simulink model "HINF4INDIFullLoop"  (R2021a)
settings: Solver=VariableStepAuto  StartTime=0.0  StopTime=50  RelTol=1e-3
values from neighbouring files (symbols this model uses):
  Ahg2 = blkdiag(Ahg2, Ahcg)    [HinFSynINDIFullLoop.m]
  Ahs3 = blkdiag(Ahs3, Ahcs)    [HinFSynINDIFullLoop.m]
  Ahs7 = blkdiag(Ahs7, Ahcs)    [HinFSynINDIFullLoop.m]
  Amc = d2c(Amd,'tustin')    [HinFSynINDIFullLoop.m]
  Asc = d2c(Asd,'tustin')    [HinFSynINDIFullLoop.m]
  Bhg2 = blkdiag(Bhg2, Bhcg)    [HinFSynINDIFullLoop.m]
  Bhs3 = blkdiag(Bhs3, Bhcs)    [HinFSynINDIFullLoop.m]
  Bhs7 = blkdiag(Bhs7, Bhcs)    [HinFSynINDIFullLoop.m]
  Chg2 = blkdiag(Chg2, Chcg)    [HinFSynINDIFullLoop.m]
  Chs3 = blkdiag(Chs3, Chcs)    [HinFSynINDIFullLoop.m]
  Chs7 = blkdiag(Chs7, Chcs)    [HinFSynINDIFullLoop.m]
  Dhg2 = blkdiag(Dhg2, Dhcg)    [HinFSynINDIFullLoop.m]
  Dhs3 = blkdiag(Dhs3, Dhcs)    [HinFSynINDIFullLoop.m]
  Dhs7 = blkdiag(Dhs7, Dhcs)    [HinFSynINDIFullLoop.m]
  Gs = [-10.67  10.67  0     0     0     0 0 ... (first row only)    [HinFSynINDIFullLoop.m]
  Gs_inv = pinv(Gs)    [HinFSynINDIFullLoop.m]
  Kdg = diag([2.0; 1.8])    [HinFSynINDIFullLoop.m]
  Kds = [10; 18; 18]    [HinFSynINDIFullLoop.m]
  Kps = [4.1089; 4.7304; 7.36]    [HinFSynINDIFullLoop.m]
  W1 = kw1*tf(numW1,denW1)    [HinFSynINDIFullLoop.m]
  W2 = kw2*tf(numW2,denW2)    [HinFSynINDIFullLoop.m]
settings Model: Creator=AutomZ2-RG02A02  LastModifiedBy=AutomZ2-RG02A02
settings SolverCC: AlgebraicLoopSolver=TrustRegion

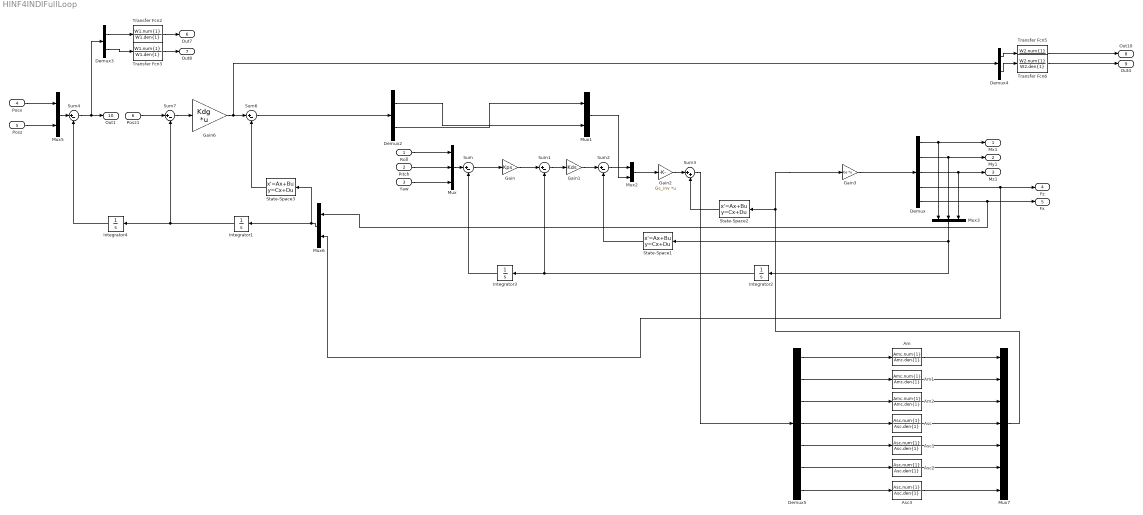
== system HINF4INDIFullLoop ==
  Roll : Inport
  Pitch : Inport  Port=2
  Yaw : Inport  Port=3
  Posx : Inport  Port=4
  Posz : Inport  Port=5
  Posz1 : Inport  Port=6  PortDimensions=2
  Am : TransferFcn  Numerator=Amc.num{1}  Denominator=Amc.den{1}
  Am1 : TransferFcn  Numerator=Amc.num{1}  Denominator=Amc.den{1}
  Am2 : TransferFcn  Numerator=Amc.num{1}  Denominator=Amc.den{1}
  Asc{,1..3} (4 alike) : TransferFcn  Numerator=Asc.num{1}  Denominator=Asc.den{1}
  Demux : Demux  Outputs=5
  Demux2 : Demux  Outputs=2
  Demux3 : Demux  Outputs=2
  Demux4 : Demux  Outputs=2
  Demux5 : Demux  Outputs=7
  Gain : Gain  Gain=Kps
  Gain1 : Gain  Gain=Kds
  Gain2 : Gain  Gain=Gs_inv  Multiplication=Matrix(K*u)
  Gain3 : Gain  Gain=Gs  Multiplication=Matrix(K*u)
  Gain6 : Gain  Gain=Kdg  Multiplication=Matrix(K*u)
  Integrator{1..4} (4 alike) : Integrator
  Mux : Mux  Inputs=3
  Mux1 : Mux  Inputs=2
  Mux2 : Mux  Inputs=[3 2]
  Mux3 : Mux  Inputs=3
  Mux5 : Mux  Inputs=2
  Mux6 : Mux  Inputs=2
  Mux7 : Mux  Inputs=7
  State-Space1 : StateSpace  A=Ahs3  B=Bhs3  C=Chs3  D=Dhs3  InitialCondition=0
  State-Space2 : StateSpace  A=Ahs7  B=Bhs7  C=Chs7  D=Dhs7  InitialCondition=0
  State-Space3 : StateSpace  A=Ahg2  B=Bhg2  C=Chg2  D=Dhg2  InitialCondition=0
  Sum{,1..2,4,6..7} (6 alike) : Sum  Inputs=|+-
  Sum3 : Sum  Inputs=|++
  Transfer Fcn2 : TransferFcn  Numerator=W1.num{1}  Denominator=W1.den{1}
  Transfer Fcn3 : TransferFcn  Numerator=W1.num{1}  Denominator=W1.den{1}
  Transfer Fcn5 : TransferFcn  Numerator=W2.num{1}  Denominator=W2.den{1}
  Transfer Fcn6 : TransferFcn  Numerator=W2.num{1}  Denominator=W2.den{1}
  Mx1 : Outport
  My1 : Outport  Port=2
  Mz1 : Outport  Port=3
  Fz : Outport  Port=4
  Fx : Outport  Port=5
  Out7 : Outport  Port=6
  Out8 : Outport  Port=7
  Out10 : Outport  Port=8
  Out4 : Outport  Port=9
  Out1 : Outport  Port=10
  wires:
  State-Space1/1 -> Sum2/2
  Mux7/1 -> Gain3/1, State-Space2/1
  Mux/1 -> Sum/1
  Mux3/1 -> State-Space1/1, Integrator2/1
  Sum1/1 -> Gain1/1
  State-Space2/1 -> Sum3/2
  Integrator2/1 -> Sum1/2, Integrator3/1
  Sum2/1 -> Mux2/1
  Mux1/1 -> Mux2/2
  Roll/1 -> Mux/1
  Gain2/1 -> Sum3/1
  Demux/2 -> Mux3/2, My1/1
  Demux/3 -> Mz1/1, Mux3/3
  Gain/1 -> Sum1/1
  Mux2/1 -> Gain2/1
  Pitch/1 -> Mux/2
  Demux/1 -> Mux3/1, Mx1/1
  Yaw/1 -> Mux/3
  Sum/1 -> Gain/1
  Integrator3/1 -> Sum/2
  Gain1/1 -> Sum2/1
  Gain3/1 -> Demux/1
  Mux6/1 -> Integrator1/1, State-Space3/1
  Integrator1/1 -> Integrator4/1, Sum7/2
  Demux/5 -> Mux6/1, Fx/1
  Sum7/1 -> Gain6/1
  Posx/1 -> Mux5/1
  Gain6/1 -> Demux4/1, Sum6/1
  Demux/4 -> Mux6/2, Fz/1
  Mux5/1 -> Sum4/1
  Posz1/1 -> Sum7/1
  Integrator4/1 -> Sum4/2
  Sum6/1 -> Demux2/1
  State-Space3/1 -> Sum6/2
  Posz/1 -> Mux5/2
  Transfer Fcn3/1 -> Out8/1
  Demux3/2 -> Transfer Fcn3/1
  Sum4/1 -> Out1/1, Demux3/1
  Transfer Fcn2/1 -> Out7/1
  Demux3/1 -> Transfer Fcn2/1
  Demux4/2 -> Transfer Fcn6/1
  Demux4/1 -> Transfer Fcn5/1
  Transfer Fcn6/1 -> Out4/1
  Transfer Fcn5/1 -> Out10/1
  Demux5/6 -> Asc2/1
  Demux5/1 -> Am/1
  Am2/1 -> Mux7/3
  Sum3/1 -> Demux5/1
  Asc3/1 -> Mux7/7
  Asc2/1 -> Mux7/6
  Am/1 -> Mux7/1
  Am1/1 -> Mux7/2
  Demux5/5 -> Asc1/1
  Demux5/7 -> Asc3/1
  Asc/1 -> Mux7/4
  Demux5/2 -> Am1/1
  Demux5/4 -> Asc/1
  Demux5/3 -> Am2/1
  Asc1/1 -> Mux7/5
  Demux2/2 -> Mux1/1
  Demux2/1 -> Mux1/2
